simulink model "helicoptertemplate_lqr_simulation"  (R2021b)
settings: Solver=ode45  StartTime=0.0  StopTime=Tsim  RelTol=1e-3
InitFcn:
  | hwinit
values from neighbouring files (symbols this model uses):
  h = 0.01    [LQR_LQI_init.m]
  sysd = c2d(sys, h)    [LQR_LQI_init.m]
undefined symbols (not defined in the file or in its folder): Kd
libraries: eeGeneralControl x1, eeLuenbergerObserver x1
settings Model: Creator=fkzhang  LastModifiedBy=rjvanderhorst
settings SolverCC: AlgebraicLoopSolver=TrustRegion
settings DataIOCC: LimitDataPoints=on  SaveFormat=Array  ReturnWorkspaceOutputs=off
settings OptimizationCC: BlockReduction=off  BooleanDataType=off  LifeSpan=inf
settings DebuggingCC: SaveWithParameterizedLinksMsg=none  UnderspecifiedInitializationDetection=Classic  MergeDetectMultiDrivingBlocksExec=none  SignalResolutionControl=TryResolveAllWithWarning  AllowSymbolicDim=off  SFUnexpectedBacktrackingDiag=warning  SFNoUnconditionalDefaultTransitionDiag=warning  SFExecutionAtInitializationDiag=none  SFMachineParentedDataDiag=warning  ArithmeticOperatorsInVariantConditions=warning
settings HardwareCC: ProdBitPerPointer=32  ProdBitPerSizeT=32  ProdBitPerPtrDiffT=32  ProdLargestAtomicFloat=None  ProdIntDivRoundTo=Undefined  ProdEndianess=Unspecified  ProdWordSize=32  ProdHWDeviceType=32-bit Generic  TargetUnknown=on
settings ModelReferenceCC: PropagateSignalLabelsOutOfModel=off
settings SFSimCC: SimUseLocalCustomCode=off  CustomCodeUndefinedFunction=UseInterfaceOnly
settings RTWCC: RTWUseLocalCustomCode=off
settings CodeAppCC: StateflowObjectComments=on
settings GRTTargetCC: TargetLangStandard=C89/C90 (ANSI)
settings ConfigComp: CovMetricSettings=dw  CovSaveCumulativeToWorkspaceVar=on  CovSaveSingleToWorkspaceVar=on  CovExternalEMLEnable=off  CovSFcnEnable=off

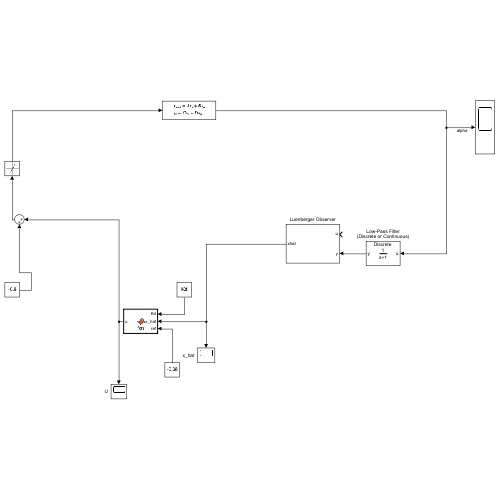
[thumbnail: Simulink's stored preview of the top-level diagram]
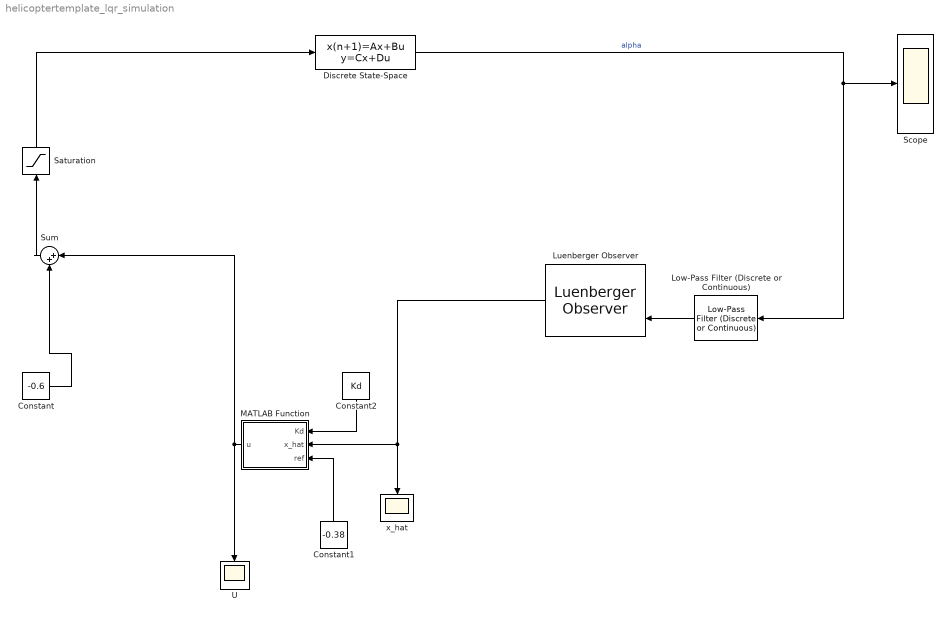
== system helicoptertemplate_lqr_simulation ==
  Constant : Constant  Value=-0.6
  Constant1 : Constant  Value=-0.38
  Constant2 : Constant  Value=Kd  LockScale=on
  Discrete State-Space : DiscreteStateSpace  A=sysd.A  B=sysd.B  C=sysd.C  D=sysd.D  SampleTime=-1
  Low-Pass Filter (Discrete or Continuous) : eeGeneralControl/Low-Pass Filter (Discrete or Continuous)  K=1  T=1  B=inf  A=-inf  init_option=Inherited from block input  x0=0  Ts=-1
  Luenberger Observer : eeLuenbergerObserver/Luenberger Observer  StateSpaceType=Discrete-time  Ad=sysd.A  Bd=sysd.B  Cd=sysd.C  Dd=sysd.D  A=1  B=1  C=1  D=1  ObserverDesign=Desired eigenvalues  Ld=2  DesiredEigenvalues=[-0.9, -0.1]  x0=[0;0]  Tsd=0.1  Ts=h
      settings: SourceProductBaseCode=PS
  MATLAB Function : MATLAB Function  TreatAsAtomicUnit=on
  Saturation : Saturate  UpperLimit=0  LowerLimit=-1
  Scope : Scope
  Sum : Sum  Inputs=|++
  U : Scope
  x_hat : Scope
  wires:
  Discrete State-Space/1 -> Scope/1, Low-Pass Filter (Discrete or Continuous)/1  "alpha"
  Low-Pass Filter (Discrete or Continuous)/1 -> Luenberger Observer/2
  Constant/1 -> Sum/2
  Sum/1 -> Saturation/1
  Saturation/1 -> Discrete State-Space/1
  Constant1/1 -> MATLAB Function/3(ref)
  MATLAB Function/1(u) -> Sum/1, U/1
  Luenberger Observer/1 -> x_hat/1, MATLAB Function/2(x_hat)
  Constant2/1 -> MATLAB Function/1(Kd)

== matlab function helicoptertemplate_lqr_simulation/MATLAB Function ==
  data: Kd input; x_hat input; u output; ref input
function u = fcn(Kd, x_hat, ref)
    x_ref = [ref; 0];
    error = x_hat-x_ref;
    u = (-Kd'*error);
end
